simulink model "cohete_modelo_simulink"  (R2018a)
settings: Solver=VariableStepAuto  StartTime=0.0  StopTime=600  FixedStep=0.00001  RelTol=1e-3
undefined symbols (not defined in the file or in its folder): ing
libraries: simulink x5
settings Model: Creator=catalina  LastModifiedBy=catalina
settings SolverCC: ZeroCrossAlgorithm=Adaptive
settings DataIOCC: Refine=1000
settings DebuggingCC: IgnoredZcDiagnostic=none

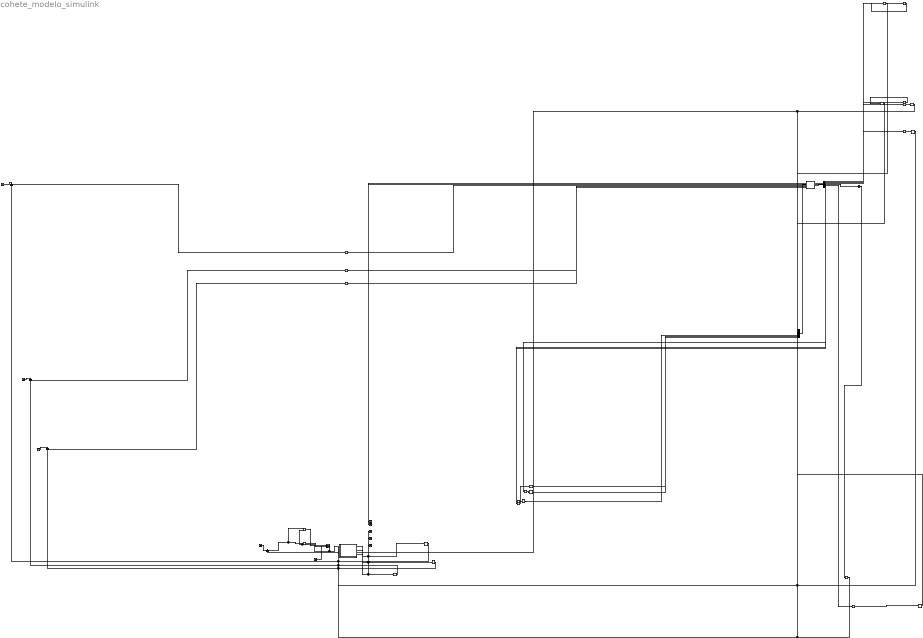
== system cohete_modelo_simulink ==
  Demux : Demux  Outputs=9
  Integrator : Integrator  InitialCondition=63/2  UpperSaturationLimit=ing
  Integrator{1,4..8} (6 alike) : Integrator  InitialCondition=0.001  UpperSaturationLimit=ing
  Integrator2 : Integrator  InitialCondition=2000  UpperSaturationLimit=ing
  Integrator3 : Integrator  InitialCondition=90*pi/180  UpperSaturationLimit=ing
  MATLAB Function : MATLAB Function  TreatAsAtomicUnit=on
  MATLAB Function1 : MATLAB Function  TreatAsAtomicUnit=on
  PID Controller : simulink/Continuous/PID Controller  Controller=PID  TimeDomain=Continuous-time  SampleTime=-1  IntegratorMethod=Forward Euler  FilterMethod=Forward Euler  Form=Parallel  UseFilter=on  ControllerParametersSource=internal  P=0.010245  I=0.034973  D=0.15114  N=3  InitialConditionSource=internal  InitialConditionForIntegrator=0  InitialConditionForFilter=0  ExternalReset=none  LimitOutput=on  UpperSaturationLimit=10  LowerSaturationLimit=-10  LinearizeAsGain=on  AntiWindupMode=back-calculation  Kb=1  TrackingMode=off  Kt=1  PParamMin=[]  PParamMax=[]  IParamMin=[]  IParamMax=[]  DParamMin=[]  DParamMax=[]  NParamMin=[]  NParamMax=[]  KbParamMin=[]  KbParamMax=[]  KtParamMin=[]  KtParamMax=[]  POutMin=[]  POutMax=[]  IOutMin=[]  IOutMax=[]  DOutMin=[]  DOutMax=[]  NOutMin=[]  NOutMax=[]  KbOutMin=[]  KbOutMax=[]  KtOutMin=[]  KtOutMax=[]  IntegratorOutMin=[]  IntegratorOutMax=[]  FilterOutMin=[]  FilterOutMax=[]  SumOutMin=[]  SumOutMax=[]  SumI1OutMin=[]  SumI1OutMax=[]  SumI2OutMin=[]  SumI2OutMax=[]  SumI3OutMin=[]  SumI3OutMax=[]  SumDOutMin=[]  SumDOutMax=[]  SaturationOutMin=[]  SaturationOutMax=[]  IntegratorContinuousStateAttributes=''  IntegratorStateMustResolveToSignalObject=off  IntegratorRTWStateStorageClass=Auto  FilterContinuousStateAttributes=''  FilterStateMustResolveToSignalObject=off  FilterRTWStateStorageClass=Auto  DifferentiatorICPrevScaledInput=0  DifferentiatorOutMin=[]  DifferentiatorOutMax=[]  FilterDiffOutCoefMin=[]  FilterDiffOutCoefMax=[]  SumDenOutMin=[]  SumDenOutMax=[]  SumNumOutMin=[]  SumNumOutMax=[]  ReciprocalOutMin=[]  ReciprocalOutMax=[]  DivideOutMin=[]  DivideOutMax=[]  TunerSelectOption=Frequency Response Based
  PID Controller1 : simulink/Continuous/PID Controller  Controller=PID  TimeDomain=Continuous-time  SampleTime=-1  IntegratorMethod=Forward Euler  FilterMethod=Forward Euler  Form=Parallel  UseFilter=on  ControllerParametersSource=internal  P=-1.1408e-06  I=-3.4583e-06  D=-1.5077e-05  N=3  InitialConditionSource=internal  InitialConditionForIntegrator=0  InitialConditionForFilter=0  ExternalReset=none  LimitOutput=on  UpperSaturationLimit=0.0052  LowerSaturationLimit=-0.0052  LinearizeAsGain=on  AntiWindupMode=back-calculation  Kb=1  TrackingMode=off  Kt=1  PParamMin=[]  PParamMax=[]  IParamMin=[]  IParamMax=[]  DParamMin=[]  DParamMax=[]  NParamMin=[]  NParamMax=[]  KbParamMin=[]  KbParamMax=[]  KtParamMin=[]  KtParamMax=[]  POutMin=[]  POutMax=[]  IOutMin=[]  IOutMax=[]  DOutMin=[]  DOutMax=[]  NOutMin=[]  NOutMax=[]  KbOutMin=[]  KbOutMax=[]  KtOutMin=[]  KtOutMax=[]  IntegratorOutMin=[]  IntegratorOutMax=[]  FilterOutMin=[]  FilterOutMax=[]  SumOutMin=[]  SumOutMax=[]  SumI1OutMin=[]  SumI1OutMax=[]  SumI2OutMin=[]  SumI2OutMax=[]  SumI3OutMin=[]  SumI3OutMax=[]  SumDOutMin=[]  SumDOutMax=[]  SaturationOutMin=[]  SaturationOutMax=[]  IntegratorContinuousStateAttributes=''  IntegratorStateMustResolveToSignalObject=off  IntegratorRTWStateStorageClass=Auto  FilterContinuousStateAttributes=''  FilterStateMustResolveToSignalObject=off  FilterRTWStateStorageClass=Auto  DifferentiatorICPrevScaledInput=0  DifferentiatorOutMin=[]  DifferentiatorOutMax=[]  FilterDiffOutCoefMin=[]  FilterDiffOutCoefMax=[]  SumDenOutMin=[]  SumDenOutMax=[]  SumNumOutMin=[]  SumNumOutMax=[]  ReciprocalOutMin=[]  ReciprocalOutMax=[]  DivideOutMin=[]  DivideOutMax=[]  TunerSelectOption=Transfer Function Based (PID Tuner App)
  PID Controller2 : simulink/Continuous/PID Controller  Controller=PID  TimeDomain=Continuous-time  SampleTime=-1  IntegratorMethod=Forward Euler  FilterMethod=Forward Euler  Form=Parallel  UseFilter=on  ControllerParametersSource=internal  P=0  I=8.6998e-05  D=0.00035383  N=3  InitialConditionSource=internal  InitialConditionForIntegrator=0  InitialConditionForFilter=0  ExternalReset=none  LimitOutput=on  UpperSaturationLimit=0.0052  LowerSaturationLimit=-0.0052  LinearizeAsGain=on  AntiWindupMode=back-calculation  Kb=1  TrackingMode=off  Kt=1  PParamMin=[]  PParamMax=[]  IParamMin=[]  IParamMax=[]  DParamMin=[]  DParamMax=[]  NParamMin=[]  NParamMax=[]  KbParamMin=[]  KbParamMax=[]  KtParamMin=[]  KtParamMax=[]  POutMin=[]  POutMax=[]  IOutMin=[]  IOutMax=[]  DOutMin=[]  DOutMax=[]  NOutMin=[]  NOutMax=[]  KbOutMin=[]  KbOutMax=[]  KtOutMin=[]  KtOutMax=[]  IntegratorOutMin=[]  IntegratorOutMax=[]  FilterOutMin=[]  FilterOutMax=[]  SumOutMin=[]  SumOutMax=[]  SumI1OutMin=[]  SumI1OutMax=[]  SumI2OutMin=[]  SumI2OutMax=[]  SumI3OutMin=[]  SumI3OutMax=[]  SumDOutMin=[]  SumDOutMax=[]  SaturationOutMin=[]  SaturationOutMax=[]  IntegratorContinuousStateAttributes=''  IntegratorStateMustResolveToSignalObject=off  IntegratorRTWStateStorageClass=Auto  FilterContinuousStateAttributes=''  FilterStateMustResolveToSignalObject=off  FilterRTWStateStorageClass=Auto  DifferentiatorICPrevScaledInput=0  DifferentiatorOutMin=[]  DifferentiatorOutMax=[]  FilterDiffOutCoefMin=[]  FilterDiffOutCoefMax=[]  SumDenOutMin=[]  SumDenOutMax=[]  SumNumOutMin=[]  SumNumOutMax=[]  ReciprocalOutMin=[]  ReciprocalOutMax=[]  DivideOutMin=[]  DivideOutMax=[]  TunerSelectOption=Transfer Function Based (PID Tuner App)
  PID Controller3 : simulink/Continuous/PID Controller  Controller=PID  TimeDomain=Continuous-time  SampleTime=-1  IntegratorMethod=Forward Euler  FilterMethod=Forward Euler  Form=Parallel  UseFilter=on  ControllerParametersSource=internal  P=0  I=754783756331.3737  D=0  N=100  InitialConditionSource=internal  InitialConditionForIntegrator=0  InitialConditionForFilter=0  ExternalReset=none  LimitOutput=on  UpperSaturationLimit=500  LowerSaturationLimit=-500  LinearizeAsGain=on  AntiWindupMode=back-calculation  Kb=1  TrackingMode=on  Kt=1  PParamMin=[]  PParamMax=[]  IParamMin=[]  IParamMax=[]  DParamMin=[]  DParamMax=[]  NParamMin=[]  NParamMax=[]  KbParamMin=[]  KbParamMax=[]  KtParamMin=[]  KtParamMax=[]  POutMin=[]  POutMax=[]  IOutMin=[]  IOutMax=[]  DOutMin=[]  DOutMax=[]  NOutMin=[]  NOutMax=[]  KbOutMin=[]  KbOutMax=[]  KtOutMin=[]  KtOutMax=[]  IntegratorOutMin=[]  IntegratorOutMax=[]  FilterOutMin=[]  FilterOutMax=[]  SumOutMin=[]  SumOutMax=[]  SumI1OutMin=[]  SumI1OutMax=[]  SumI2OutMin=[]  SumI2OutMax=[]  SumI3OutMin=[]  SumI3OutMax=[]  SumDOutMin=[]  SumDOutMax=[]  SaturationOutMin=[]  SaturationOutMax=[]  IntegratorContinuousStateAttributes=''  IntegratorStateMustResolveToSignalObject=off  IntegratorRTWStateStorageClass=Auto  FilterContinuousStateAttributes=''  FilterStateMustResolveToSignalObject=off  FilterRTWStateStorageClass=Auto  DifferentiatorICPrevScaledInput=0  DifferentiatorOutMin=[]  DifferentiatorOutMax=[]  FilterDiffOutCoefMin=[]  FilterDiffOutCoefMax=[]  SumDenOutMin=[]  SumDenOutMax=[]  SumNumOutMin=[]  SumNumOutMax=[]  ReciprocalOutMin=[]  ReciprocalOutMax=[]  DivideOutMin=[]  DivideOutMax=[]  TunerSelectOption=Frequency Response Based
  PID Controller4 : simulink/Continuous/PID Controller  Controller=PID  TimeDomain=Continuous-time  SampleTime=-1  IntegratorMethod=Forward Euler  FilterMethod=Forward Euler  Form=Parallel  UseFilter=on  ControllerParametersSource=internal  P=0  I=-565.1956  D=-130323.6169  N=30  InitialConditionSource=internal  InitialConditionForIntegrator=0  InitialConditionForFilter=0  ExternalReset=none  LimitOutput=on  UpperSaturationLimit=1000  LowerSaturationLimit=-1000  LinearizeAsGain=on  AntiWindupMode=back-calculation  Kb=1  TrackingMode=on  Kt=1  PParamMin=[]  PParamMax=[]  IParamMin=[]  IParamMax=[]  DParamMin=[]  DParamMax=[]  NParamMin=[]  NParamMax=[]  KbParamMin=[]  KbParamMax=[]  KtParamMin=[]  KtParamMax=[]  POutMin=[]  POutMax=[]  IOutMin=[]  IOutMax=[]  DOutMin=[]  DOutMax=[]  NOutMin=[]  NOutMax=[]  KbOutMin=[]  KbOutMax=[]  KtOutMin=[]  KtOutMax=[]  IntegratorOutMin=[]  IntegratorOutMax=[]  FilterOutMin=[]  FilterOutMax=[]  SumOutMin=[]  SumOutMax=[]  SumI1OutMin=[]  SumI1OutMax=[]  SumI2OutMin=[]  SumI2OutMax=[]  SumI3OutMin=[]  SumI3OutMax=[]  SumDOutMin=[]  SumDOutMax=[]  SaturationOutMin=[]  SaturationOutMax=[]  IntegratorContinuousStateAttributes=''  IntegratorStateMustResolveToSignalObject=off  IntegratorRTWStateStorageClass=Auto  FilterContinuousStateAttributes=''  FilterStateMustResolveToSignalObject=off  FilterRTWStateStorageClass=Auto  DifferentiatorICPrevScaledInput=0  DifferentiatorOutMin=[]  DifferentiatorOutMax=[]  FilterDiffOutCoefMin=[]  FilterDiffOutCoefMax=[]  SumDenOutMin=[]  SumDenOutMax=[]  SumNumOutMin=[]  SumNumOutMax=[]  ReciprocalOutMin=[]  ReciprocalOutMax=[]  DivideOutMin=[]  DivideOutMax=[]  TunerSelectOption=Frequency Response Based
  Scope{,1..4} (5 alike) : Scope
  Step : Step  After=1000  SampleTime=0
  Step1 : Step  After=10000  SampleTime=0
  Step2 : Step  After=1000  SampleTime=0
  Step3 : Step  Before=10  After=0  SampleTime=0
  Step4 : Step  Time=500  SampleTime=0
  Sum : Sum  Inputs=+-
  Sum1 : Sum  Inputs=+-
  Sum2 : Sum  Inputs=+-
  Sum3 : Sum  Inputs=|+-
  Switch : Switch  Threshold=500
  Transport Delay{,1,3..11} (11 alike) : TransportDelay
  Transport Delay2 : TransportDelay  InitialOutput=2000
  Vector Concatenate : Concatenate  NumInputs=9
  wires:
  MATLAB Function1/3(h) -> Transport Delay11/1, Scope2/1
  MATLAB Function1/2(y) -> Transport Delay10/1, Scope1/1
  MATLAB Function1/1(x) -> Transport Delay9/1, Scope/1
  Step/1 -> Sum/1
  Step1/1 -> Sum1/1
  Step2/1 -> Sum2/1
  Demux/1 -> Integrator/1
  Demux/2 -> Integrator1/1
  Demux/3 -> Integrator2/1
  Demux/4 -> Integrator3/1, Scope3/1
  Demux/6 -> Integrator5/1
  Demux/7 -> Integrator6/1
  Demux/8 -> Integrator7/1
  Demux/9 -> Integrator8/1
  Integrator1/1 -> Transport Delay/1
  Integrator/1 -> Transport Delay1/1
  Transport Delay1/1 -> Vector Concatenate/1
  Integrator2/1 -> Transport Delay2/1
  Transport Delay2/1 -> Sum3/2, Vector Concatenate/3
  Integrator4/1 -> Transport Delay3/1
  Transport Delay3/1 -> MATLAB Function1/3(theta), Vector Concatenate/5
  Transport Delay/1 -> Vector Concatenate/2
  Integrator3/1 -> Transport Delay4/1
  Transport Delay4/1 -> MATLAB Function1/2(phi), Vector Concatenate/4
  Integrator5/1 -> Transport Delay5/1
  Transport Delay5/1 -> Vector Concatenate/6
  Integrator6/1 -> Transport Delay6/1
  Transport Delay6/1 -> Vector Concatenate/7
  Integrator7/1 -> Transport Delay7/1
  Transport Delay7/1 -> Vector Concatenate/8
  Integrator8/1 -> Transport Delay8/1
  Transport Delay8/1 -> Vector Concatenate/9
  Transport Delay9/1 -> Sum1/2, MATLAB Function1/4(xant)
  Transport Delay10/1 -> Sum2/2, MATLAB Function1/5(yant)
  Transport Delay11/1 -> Sum/2, MATLAB Function1/6(zant)
  MATLAB Function/1(xprima) -> Demux/1
  Vector Concatenate/1 -> MATLAB Function/2(x)
  Step3/1 -> Sum3/1
  Step4/1 -> Switch/2
  Demux/5 -> Integrator4/1, Scope4/1
  PID Controller2/1 -> MATLAB Function/5(uy)
  Sum2/1 -> PID Controller2/1
  PID Controller1/1 -> MATLAB Function/4(ux)
  Sum/1 -> PID Controller1/1
  PID Controller/1 -> MATLAB Function/3(ut)
  Sum1/1 -> PID Controller/1
  PID Controller4/1 -> Switch/3
  PID Controller3/1 -> Switch/1
  Sum3/1 -> PID Controller3/1, PID Controller4/1
  Switch/1 -> MATLAB Function1/1(vel), PID Controller3/2, PID Controller4/2

== matlab function cohete_modelo_simulink/MATLAB Function1 ==
  data: vel input; x output; phi input; theta input; xant input; yant input; y output; zant input; h output
function [x, y, h]=cartesianas(vel, phi, theta, xant,yant, zant)
Ts = 0.1;

x = xant + vel*cos(phi)*cos(theta)*Ts;
y = yant + vel*cos(phi)*sin(theta)*Ts;
h = zant + vel*sin(phi)*Ts;

if h < 0
    h = 0;
end

== matlab function cohete_modelo_simulink/MATLAB Function ==
  data: t input; xprima output; x input; ut input; ux input; uy input
function xprima=cohete_modelov2(t,x,ut,ux,uy)
xprima = zeros(1,9);
g0 = 9.8065;  % gravedad (se asume constante en altura)
ro0= 0.1; % coef resistencia superficie terrestre
ve=5000; % velocidad de escape de gases
Ac=7.5; % area transversal para calculo de roce con aire
Mmin=100; % masa del cohete sin combustible

%Ruido
mu=0;
sigma=0.5*pi/180;

% maximos para tobera
utMax=10; % maximo empuje longitudinal
uxMax=0.3*pi/180;  % maxima inclinacion tobera en eje x del cohete
uyMax=0.3*pi/180;  % maxima inclinacion tobera en eje y del cohete

if x(3)<Mmin   % se acabo el combustible
    ut=0;
end

L=63; % largo cohete
Ir=x(3)*L^2/12; % momento de inercia rotacional cohete

% FUERZAS MAXIMAS
if ut>utMax, ut=utMax; end;
if ut<0, ut=0; end;


if ux>uxMax, ux=uxMax; end;
if ux<-uxMax, ux=-uxMax; end;
if uy>uyMax, uy=uyMax; end;
if uy<-uyMax, uy=-uyMax; end;


% ECUACIONES DIFERENCIALES SIMPLIFICADAS
% g=g0*(Rs/(Rs+x(1))); % gravedad
Ftob=ut*ve; % fuerza tobera empuje, thrust
Fux=Ftob*sin(x(8)); % componente de fuerza tobera transversal X
Fuy=Ftob*sin(x(9)); % componente de fuerza tobera transversal Y
Fp=sqrt((Ftob)^2-Fux^2-Fuy^2); % fuerza empuje vertical
ro=ro0*((1 - (x(1)/20000)^2)>0)*(1 - (x(1)/20000)^2); % roce aire



xprima(1)=x(2); % dh/dt
xprima(2)=(Fp - ro*Ac*sign(x(2))*abs(x(2))^(3/2)- x(3)*g0*sin(x(4)))/x(3); % dh^2/dt^2
xprima(3)=-ut; % dM/dT
xprima(4)=x(6); % d_phi/dt
xprima(5)=x(7);%+normrnd(mu,sigma); % d_theta/dt
xprima(6)=(L/2)*(Fux-1*g0*cos(x(4))-1500*x(6))/Ir;  % d^2_phi/dt^2
xprima(7)=(L/2)*(Fuy-1500*x(7))/Ir;  % d^2_theta/dt^2
xprima(8) = (ux-x(8))/2;
xprima(9) = (uy-x(9))/2;

% [x(8),xprima(8)]

% xprima=xprima';
